simulink subsystem "Circular_Port_Model"  (R2020b)
settings: Solver=VariableStepAuto  StartTime=0.0  StopTime=10.0  RelTol=1e-3
undefined symbols (not defined in the file): Sim
settings Model: Creator=Edward  LastModifiedBy=Edward

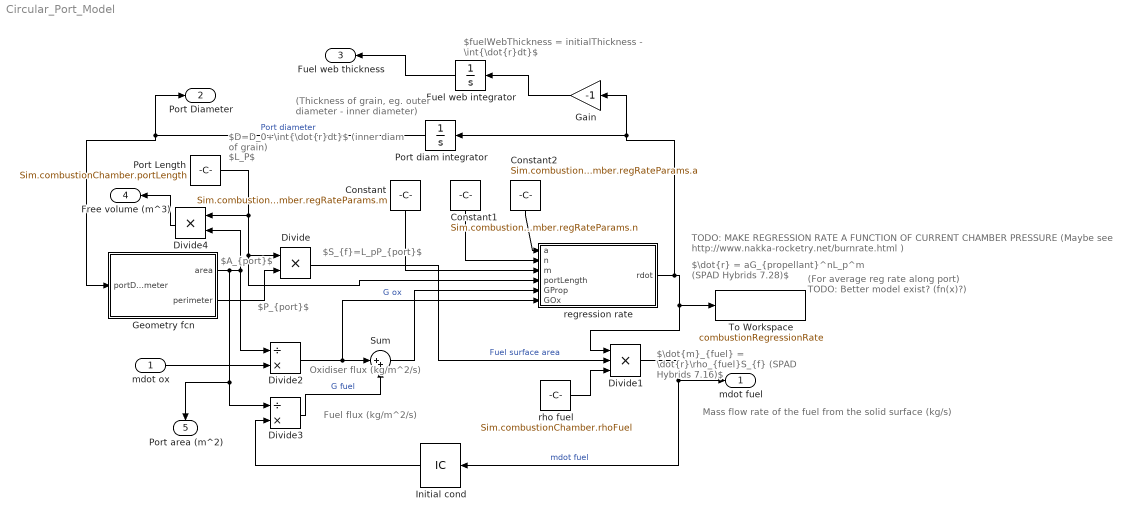
== system Circular_Port_Model ==
  note: Fuel flux (kg/m^2/s)
  note: Mass flow rate of the fuel from the solid surface (kg/s)
  note: $\dot{r} = aG_{propellant}^nL_p^m (SPAD Hybrids 7.28)$
  note: (For average reg rate along port)
      | TODO: Better model exist? (fn(x)?)
  note: $L_P$
  note: $D=D_0+\int{\dot{r}dt}$ (inner diam of grain)
  note: $fuelWebThickness = initialThickness - \int{\dot{r}dt}$
  note: (Thickness of grain, eg. outer
      | diameter - inner diameter)
  note: Oxidiser flux (kg/m^2/s)
  note: $\dot{m}_{fuel} = \dot{r}\rho_{fuel}S_{f} (SPAD Hybrids 7.16)$
  note: $P_{port}$
  note: $A_{port}$
  note: $S_{f}=L_pP_{port}$
  note: TODO: MAKE REGRESSION RATE A FUNCTION OF CURRENT CHAMBER PRESSURE (Maybe see http://www.nakka-rocketry.net/burnrate.html )
  mdot ox : Inport
  Constant : Constant  Value=Sim.combustionChamber.regRateParams.m
  Constant1 : Constant  Value=Sim.combustionChamber.regRateParams.n
  Constant2 : Constant  Value=Sim.combustionChamber.regRateParams.a
  Divide : Product  Inputs=**
  Divide1 : Product  Inputs=***
  Divide2 : Product  Inputs=/*
  Divide3 : Product  Inputs=/*
  Divide4 : Product  Inputs=**
  "Fuel web integrator " : Integrator  InitialCondition=Sim.combustionChamber.initialFuelWebThickness
  Gain : Gain  Gain=-1
  "Geometry fcn " : MATLAB Function  TreatAsAtomicUnit=on
  Initial cond : InitialCondition  Value=Sim.combustionChamber.mdotOxInitial / Sim.combustionChamber.OFRatioInitial
  Port Length : Constant  Value=Sim.combustionChamber.portLength
  Port diam integrator : Integrator  InitialCondition=Sim.combustionChamber.initialPortDiameter
  Sum : Sum  Inputs=|++
  To Workspace : ToWorkspace  VariableName=combustionRegressionRate  SaveFormat=Timeseries  SampleTime=-1
  regression rate : MATLAB Function  TreatAsAtomicUnit=on
  rho fuel : Constant  Value=Sim.combustionChamber.rhoFuel
  mdot fuel : Outport
  Port Diameter : Outport  Port=2
  Fuel web thickness : Outport  Port=3
  Free volume (m^3) : Outport  Port=4
  Port area (m^2) : Outport  Port=5
  wires:
  Divide4/1 -> Free volume (m^3)/1
  "Geometry fcn "/2(perimeter) -> Divide/2
  Initial cond/1 -> Divide3/2
  Constant2/1 -> regression rate/1(a)
  Constant1/1 -> regression rate/2(n)
  Constant/1 -> regression rate/3(m)
  "Fuel web integrator "/1 -> Fuel web thickness/1
  Gain/1 -> "Fuel web integrator "/1
  regression rate/1(rdot) -> Gain/1, Port diam integrator/1, To Workspace/1, Divide1/1
  Port diam integrator/1 -> "Geometry fcn "/1(portDiameter), Port Diameter/1  "Port diameter"
  Sum/1 -> regression rate/5(GProp)
  mdot ox/1 -> Divide2/2
  Divide2/1 -> regression rate/6(GOx), Sum/1  "G ox"
  Divide3/1 -> Sum/2  "G fuel"
  Divide1/1 -> mdot fuel/1, Initial cond/1  "mdot fuel"
  rho fuel/1 -> Divide1/3
  Divide/1 -> Divide1/2  "Fuel surface area"
  "Geometry fcn "/1(area) -> Divide3/1, Port area (m^2)/1, Divide2/1, Divide4/2
  Port Length/1 -> Divide4/1, regression rate/4(portLength), Divide/1

== matlab function Circular_Port_Model/Geometry fcn  ==
  data: portDiameter input; area output; perimeter output
function [area, perimeter] = fcn(portDiameter)
area = pi.*(portDiameter./2).^2;
perimeter = pi.*portDiameter;

== matlab function Circular_Port_Model/regression rate ==
  data: a input; n input; m input; portLength input; rdot output; GProp input; GOx input; useOxidiserFluxOnlyRegRateEquation parameter
function rdot = regressionRate(a, n, m, portLength, GProp, GOx, useOxidiserFluxOnlyRegRateEquation)

%Grosse (2009) using Sasolwax 0907 - Using GOx equation
% a = 0.132e-3;
% n = 0.555;

% %McCormick et al (2005) using FR5560 - Using GOx equation
% a = 0.155e-3;
% n = 0.5;
if(useOxidiserFluxOnlyRegRateEquation)
    rdot = a.*(GOx.^n);
else
    rdot = a.*(GProp.^n).*portLength.^m;
end
